simulink model "GOcontroll_Crank_Example"  (R2023b)
settings: Solver=FixedStepDiscrete  StartTime=0.0  StopTime=5  FixedStep=0.01  RelTol=1e-3
PreLoadFcn:
  | librarySetup
PostLoadFcn:
  | core_info = evalc('feature(''numcores'')');
  | core_info_split = split(core_info, " ");
  | num_cores = core_info_split{12};
  | set_param(bdroot, "MakeCommand", ['make_rtw -j' num_cores]);
  | clear num_cores core_info core_info_split
undefined symbols (not defined in the file): DiscIntNeverNeededParam, missing
libraries: GOcontroll_Crank x8, simulink x2
settings Model: Creator=la_obwlf  LastModifiedBy=maud
settings SolverCC: AlgebraicLoopSolver=TrustRegion
settings DataIOCC: LimitDataPoints=on  SaveFormat=Array  ReturnWorkspaceOutputs=off
settings OptimizationCC: BlockReduction=off  DefaultParameterBehavior=Inlined  LifeSpan=1  EfficientTunableParamExpr=on
settings DebuggingCC: SolverPrmCheckMsg=warning  InheritedTsInSrcMsg=none  MultiTaskRateTransMsg=warning  ParameterPrecisionLossMsg=none  UnconnectedInputMsg=warning  UnconnectedOutputMsg=warning  SFUnusedDataAndEventsDiag=none  SFUnexpectedBacktrackingDiag=warning  SFNoUnconditionalDefaultTransitionDiag=warning  SFUndirectedBroadcastEventsDiag=none  SFExecutionAtInitializationDiag=none  RCSCRenamedMsg=none  RCSCObservableMsg=none  ArithmeticOperatorsInVariantConditions=warning
settings HardwareCC: ProdBitPerLong=64  ProdLargestAtomicInteger=Long  ProdLargestAtomicFloat=Double  ProdLongLongMode=on  ProdHWDeviceType=ARM Compatible->ARM 64-bit (LP64)
settings ModelReferenceCC: EnableRefExpFcnMdlSchedulingChecks=on  PropagateSignalLabelsOutOfModel=off
settings SFSimCC: SimUseLocalCustomCode=off  MATLABDynamicMemAlloc=off  CustomCodeUndefinedFunction=UseInterfaceOnly
settings RTWCC: Description=Linux Embedded Coder  SystemTargetFile=ert_linux.tlc  MakeCommand=make_rtw -j24  TemplateMakefile=ert_linux_target_64.tmf  RetainRTWFile=on  RTWUseLocalCustomCode=off
settings CodeAppCC: IgnoreCustomStorageClasses=off  StateflowObjectComments=on
settings STFCustomTargetCC: TargetLangStandard=C89/C90 (ANSI)  CodeReplacementLibrary=GNU C99 extensions  CombineOutputUpdateFcns=on  ERTCustomFileBanners=on  SupportContinuousTime=off  SupportNonInlinedSFcns=off  RemoveResetFunc=on  MATLABClassNameForMDSCustomization=Simulink.SoftwareTarget.ERTCustomization  SystemTargetFile=ert_linux.tlc
settings ERTTargetCC: CodeReplacementLibrary=GNU C99 extensions  MultiwordLength=2048  ParMdlRefBuildCompliant=off  CompOptLevelCompliant=off  ConcurrentExecutionCompliant=off  ModelStepFunctionPrototypeControlCompliant=off  CPPClassGenCompliant=off  UseToolchainInfoCompliant=off  ERTCustomFileTemplate=ert_linux_file_process.tlc  PreserveExpressionOrder=on  SuppressUnreachableDefaultCases=off
settings ConfigComp: CovMetricSettings=dw  CovSaveCumulativeToWorkspaceVar=on  CovSaveSingleToWorkspaceVar=on  CovExternalEMLEnable=off  CovSFcnEnable=off

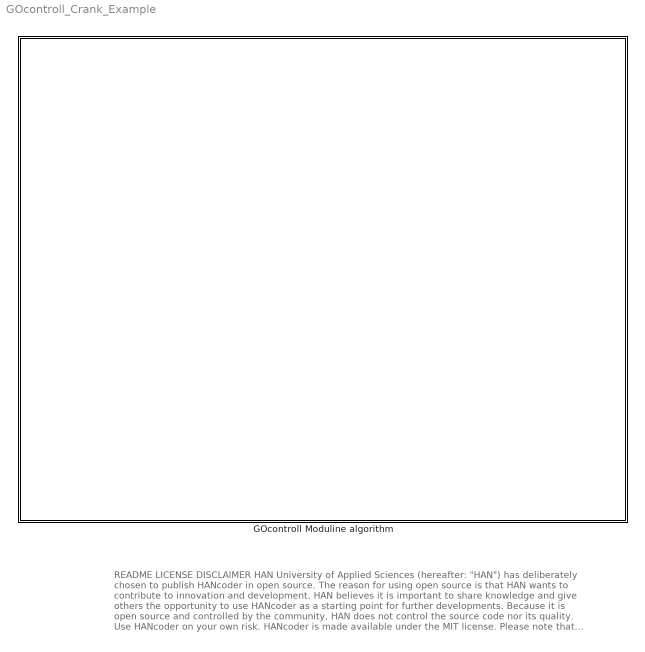
== system GOcontroll_Crank_Example ==
  note: README
      |
      | LICENSE
      |
      | DISCLAIMER
      |
      | HAN University of Applied Sciences (hereafter: "HAN") has deliberately chosen
      | to publish HANcoder in open source. The reason for using open source is that
      | HAN wants to contribute to innovation and development. HAN believes it is
      | important to share knowledge and give others the opportunity to use HANcoder
      | as a starting point for further developments. Because it is open source and
      | controlled by the community, HAN does not control the source code nor its
      | quality. Use HANcoder on your own risk. HANcoder is made available under the
      | MIT license. Please note that this license contains an exclusion of liability.
  GOcontroll Moduline algorithm : Subsystem  mask(TopLevelSubsystem){}
      mask Display: image(imread('GOcontroll.png'))

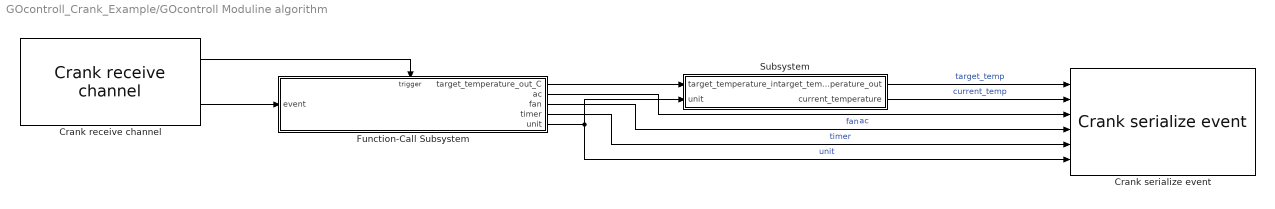
== system GOcontroll_Crank_Example/GOcontroll Moduline algorithm ==
  Crank receive channel : GOcontroll_Crank/Crank receive channel  field_names="[\"num\" \"unit\" string(missing) string(missing) string(missing) string(missing);\"num\" \"unit\" string(missing) string(missing) string(missing) string(missing);\"target_temperature\" \"current_temperature\" \"ac\" \"fan\" \"timer\" \"units\"]"  num_fields=[2 2 6 0 0 0 0]  field_types=[5 5 0 0 0 0;5 5 0 0 0 0;4 4 3 3 3 3]  fmts="[\"2u1 num 2u1 unit\" \"2u1 num 2u1 unit\" \"2s1 target_temperature 2s1 current_temperature 1u1 ac 1u1 fan 1u1 timer 1u1 units\" \"\" \"\" \"\" \"\"]"  tsamp=0.01  nbuff_len=100  channel='thermostat_backend'  header_text=|  events="[\"decrease_temperature\",\"increase_temperature\",\"thermostat_update\",\"toggle_ac\",\"toggle_fan\",\"toggle_timer\",\"toggle_units\"]"  header='ThermostatIO_events.h'  num_events=7
      | #define DECREASE_TEMPERATURE_EVENT "decrease_temperature"
      | #define DECREASE_TEMPERATURE_FMT "2u1 num 2u1 unit"
      | typedef struct {
      | 	uint16_t 		num;
      | 	uint16_t 		unit;
      | } decrease_temperature_event_t;
      | 
      | #define INCREASE_TEMPERATURE_EVENT "increase_temperature"
      | #define INCREASE_TEMPERATURE_FMT "2u1 num 2u1 unit"
      | typedef struct {
      | 	uint16_t 		num;
      | 	uint16_t 		unit;
      | } increase_temperature_event_t;
      | 
      | #define THERMOSTAT_UPDATE_EVENT "thermostat_update"
      | #define THERMOSTAT_UPDATE_FMT "2s1 target_temperature 2s1 current_temperature 1u1 ac 1u1 fan 1u1 timer 1u1 units"
      | typedef struct {
      | 	int16_t 		target_temperature;
      | 	int16_t 		current_temperature;
      | 	uint8_t 		ac;
      | 	uint8_t 		fan;
      | 	uint8_t 		timer;
      | 	uint8_t 		units;
      | } thermostat_update_event_t;
      | 
      | #define TOGGLE_AC_EVENT "toggle_ac"
      | 
      | #define TOGGLE_FAN_EVENT "toggle_fan"
      | 
      | #define TOGGLE_TIMER_EVENT "toggle_timer"
      | 
      | #define TOGGLE_UNITS_EVENT "toggle_units"
      settings: SourceProductName=GOcontroll Crank
  Crank serialize event : GOcontroll_Crank/Crank serialize event  field_types=[5 5 0 0 0 0;5 5 0 0 0 0;4 4 3 3 3 3]  tsamp=0.01  channel='thermostat_frontend'  event_name=thermostat_update  input_names="[\"target_temperature\",\"current_temperature\",\"ac\",\"fan\",\"timer\",\"units\"]"  input_datatypes=[4 4 3 3 3 3]  header='ThermostatIO_events.h'  header_text=|  num_fields=[2 2 6 0 0 0 0]  field_names="[\"num\" \"unit\" string(missing) string(missing) string(missing) string(missing);\"num\" \"unit\" string(missing) string(missing) string(missing) string(missing);\"target_temperature\" \"current_temperature\" \"ac\" \"fan\" \"timer\" \"units\"]"  fmts="[\"2u1 num 2u1 unit\" \"2u1 num 2u1 unit\" \"2s1 target_temperature 2s1 current_temperature 1u1 ac 1u1 fan 1u1 timer 1u1 units\" \"\" \"\" \"\" \"\"]"  events="[\"decrease_temperature\" \"increase_temperature\" \"thermostat_update\" \"toggle_ac\" \"toggle_fan\" \"toggle_timer\" \"toggle_units\"]"
      | #define DECREASE_TEMPERATURE_EVENT "decrease_temperature"
      | #define DECREASE_TEMPERATURE_FMT "2u1 num 2u1 unit"
      | typedef struct {
      | 	uint16_t 		num;
      | 	uint16_t 		unit;
      | } decrease_temperature_event_t;
      | 
      | #define INCREASE_TEMPERATURE_EVENT "increase_temperature"
      | #define INCREASE_TEMPERATURE_FMT "2u1 num 2u1 unit"
      | typedef struct {
      | 	uint16_t 		num;
      | 	uint16_t 		unit;
      | } increase_temperature_event_t;
      | 
      | #define THERMOSTAT_UPDATE_EVENT "thermostat_update"
      | #define THERMOSTAT_UPDATE_FMT "2s1 target_temperature 2s1 current_temperature 1u1 ac 1u1 fan 1u1 timer 1u1 units"
      | typedef struct {
      | 	int16_t 		target_temperature;
      | 	int16_t 		current_temperature;
      | 	uint8_t 		ac;
      | 	uint8_t 		fan;
      | 	uint8_t 		timer;
      | 	uint8_t 		units;
      | } thermostat_update_event_t;
      | 
      | #define TOGGLE_AC_EVENT "toggle_ac"
      | 
      | #define TOGGLE_FAN_EVENT "toggle_fan"
      | 
      | #define TOGGLE_TIMER_EVENT "toggle_timer"
      | 
      | #define TOGGLE_UNITS_EVENT "toggle_units"
      settings: SourceProductName=GOcontroll Crank
  Function-Call Subsystem : Subsystem  TreatAsAtomicUnit=on
  Subsystem : Subsystem
  wires:
  Crank receive channel/1 -> Function-Call Subsystem/Trigger
  Crank receive channel/2 -> Function-Call Subsystem/1(event)
  Function-Call Subsystem/2(ac) -> Crank serialize event/3  "ac"
  Function-Call Subsystem/3(fan) -> Crank serialize event/4  "fan"
  Function-Call Subsystem/4(timer) -> Crank serialize event/5  "timer"
  Function-Call Subsystem/5(unit) -> Subsystem/2(unit), Crank serialize event/6  "unit"
  Subsystem/2(current_temperature) -> Crank serialize event/2  "current_temp"
  Function-Call Subsystem/1(target_temperature_out_C) -> Subsystem/1(target_temperature_in)
  Subsystem/1(target_temperature_out) -> Crank serialize event/1  "target_temp"

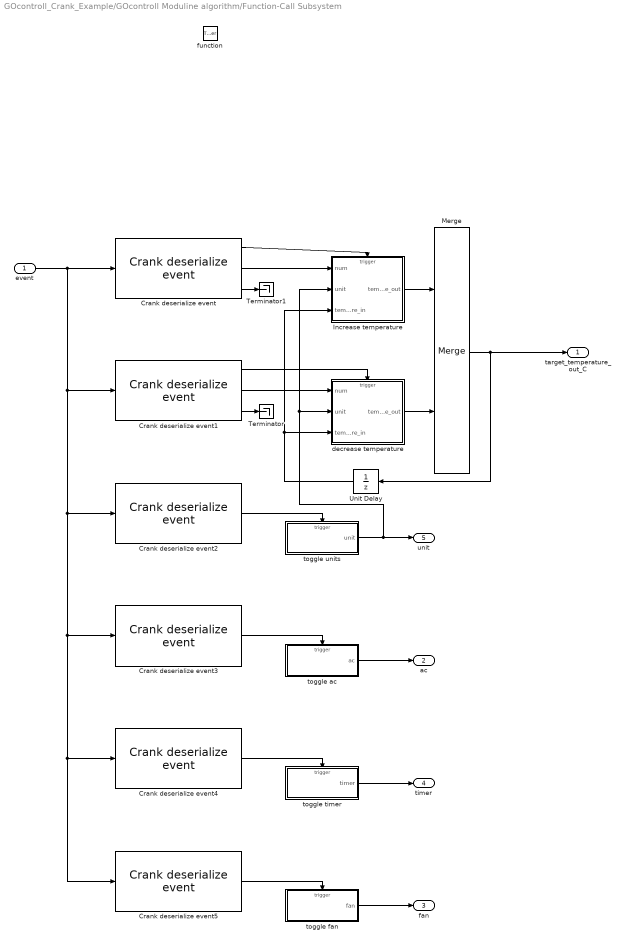
== system GOcontroll_Crank_Example/GOcontroll Moduline algorithm/Function-Call Subsystem ==
  event : Inport
  function : TriggerPort  TriggerType=function-call  VariantControl=(inherit)
  Crank deserialize event : GOcontroll_Crank/Crank deserialize event  channel='thermostat_backend'  event_name=increase_temperature  event_num=1  output_names="[\"num\",\"unit\"]"  output_datatypes=[5 5]
      settings: SourceProductName=GOcontroll Crank
  Crank deserialize event1 : GOcontroll_Crank/Crank deserialize event  channel='thermostat_backend'  event_name=decrease_temperature  event_num=0  output_names="[\"num\",\"unit\"]"  output_datatypes=[5 5]
      settings: SourceProductName=GOcontroll Crank
  Crank deserialize event2 : GOcontroll_Crank/Crank deserialize event  channel='thermostat_backend'  event_name=toggle_units  event_num=6  output_names=[]  output_datatypes=[]
      settings: SourceProductName=GOcontroll Crank
  Crank deserialize event3 : GOcontroll_Crank/Crank deserialize event  channel='thermostat_backend'  event_name=toggle_ac  event_num=3  output_names=[]  output_datatypes=[]
      settings: SourceProductName=GOcontroll Crank
  Crank deserialize event4 : GOcontroll_Crank/Crank deserialize event  channel='thermostat_backend'  event_name=toggle_timer  event_num=5  output_names=[]  output_datatypes=[]
      settings: SourceProductName=GOcontroll Crank
  Crank deserialize event5 : GOcontroll_Crank/Crank deserialize event  channel='thermostat_backend'  event_name=toggle_fan  event_num=4  output_names=[]  output_datatypes=[]
      settings: SourceProductName=GOcontroll Crank
  Increase temperature : Subsystem  TreatAsAtomicUnit=on
  Merge : Merge  InitialOutput=single(16)
  Terminator : Terminator
  Terminator1 : Terminator
  Unit Delay : UnitDelay  InitialCondition=single(16)  SampleTime=-1  HasFrameUpgradeWarning=on
  decrease temperature : Subsystem  TreatAsAtomicUnit=on
  toggle ac : Subsystem  TreatAsAtomicUnit=on
  toggle fan : Subsystem  TreatAsAtomicUnit=on
  toggle timer : Subsystem  TreatAsAtomicUnit=on
  toggle units : Subsystem  TreatAsAtomicUnit=on
  target_temperature_out_C : Outport
  ac : Outport  Port=2
  fan : Outport  Port=3
  timer : Outport  Port=4
  unit : Outport  Port=5
  wires:
  event/1 -> Crank deserialize event5/1, Crank deserialize event4/1, Crank deserialize event3/1, Crank deserialize event2/1, Crank deserialize event1/1, Crank deserialize event/1
  Crank deserialize event/2 -> Increase temperature/1(num)
  Crank deserialize event/1 -> Increase temperature/Trigger
  Crank deserialize event1/1 -> decrease temperature/Trigger
  Crank deserialize event1/2 -> decrease temperature/1(num)
  decrease temperature/1(temperature_out) -> Merge/2
  Increase temperature/1(temperature_out) -> Merge/1
  Crank deserialize event2/1 -> toggle units/Trigger
  toggle units/1(unit) -> Increase temperature/2(unit), decrease temperature/2(unit), unit/1
  Crank deserialize event3/1 -> toggle ac/Trigger
  toggle ac/1(ac) -> ac/1
  toggle timer/1(timer) -> timer/1
  Crank deserialize event4/1 -> toggle timer/Trigger
  Crank deserialize event5/1 -> toggle fan/Trigger
  toggle fan/1(fan) -> fan/1
  Unit Delay/1 -> Increase temperature/3(temperature_in), decrease temperature/3(temperature_in)
  Merge/1 -> Unit Delay/1, target_temperature_out_C/1
  Crank deserialize event1/3 -> Terminator/1
  Crank deserialize event/3 -> Terminator1/1

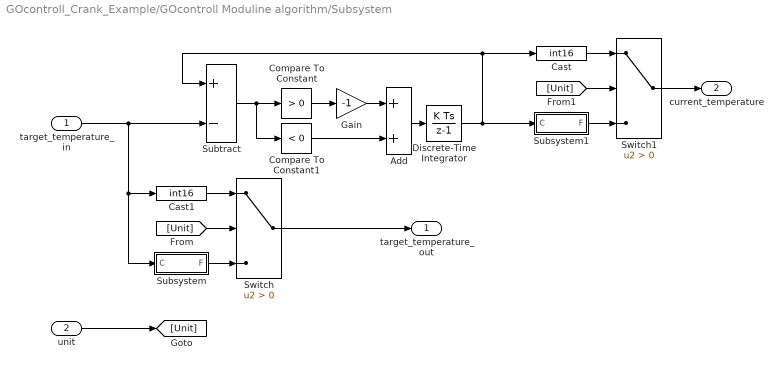
== system GOcontroll_Crank_Example/GOcontroll Moduline algorithm/Subsystem ==
  target_temperature_in : Inport
  unit : Inport  Port=2
  Add : Sum  OutDataTypeStr=int16  AccumDataTypeStr=int16
  Cast : DataTypeConversion  OutDataTypeStr=int16  SaturateOnIntegerOverflow=off  RndMeth=Floor
  Cast1 : DataTypeConversion  OutDataTypeStr=int16  SaturateOnIntegerOverflow=off  RndMeth=Floor
  Compare To Constant : simulink/Logic and Bit Operations/Compare To Constant  relop=>  const=0  OutDataTypeStr=uint8
  Compare To Constant1 : simulink/Logic and Bit Operations/Compare To Constant  relop=<  const=0  OutDataTypeStr=uint8
  Discrete-Time Integrator : DiscreteIntegrator  gainval=0.5  InitialCondition=16  SampleTime=2  OutDataTypeStr=single  ICPrevOutput=DiscIntNeverNeededParam  ICPrevScaledInput=DiscIntNeverNeededParam
  Gain : Gain  Gain=-1  ParamDataTypeStr=int16  OutDataTypeStr=single
  Subsystem : Subsystem
  Subsystem1 : Subsystem
  Subtract : Sum  Inputs=+-
  Switch : Switch  Criteria=u2 > Threshold  SaturateOnIntegerOverflow=off  InputSameDT=off
  Switch1 : Switch  Criteria=u2 > Threshold  SaturateOnIntegerOverflow=off  InputSameDT=off
  target_temperature_out : Outport
  current_temperature : Outport  Port=2
  wires:
  Subtract/1 -> Compare To Constant1/1, Compare To Constant/1
  Compare To Constant/1 -> Gain/1
  Gain/1 -> Add/1
  Compare To Constant1/1 -> Add/2
  Add/1 -> Discrete-Time Integrator/1
  Switch/1 -> target_temperature_out/1
  Subsystem/1(F) -> Switch/3
  target_temperature_in/1 -> Subsystem/1(C), Cast1/1, Subtract/2
  [Unit] -> Switch/2
  unit/1 -> [Unit]
  [Unit] -> Switch1/2
  Discrete-Time Integrator/1 -> Subsystem1/1(C), Cast/1, Subtract/1
  Subsystem1/1(F) -> Switch1/3
  Switch1/1 -> current_temperature/1
  Cast/1 -> Switch1/1
  Cast1/1 -> Switch/1

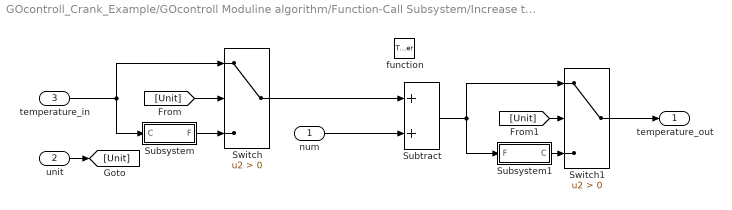
== system GOcontroll_Crank_Example/GOcontroll Moduline algorithm/Function-Call Subsystem/Increase temperature ==
  num : Inport
  unit : Inport  Port=2
  temperature_in : Inport  Port=3  Unit=degC
  function : TriggerPort  TriggerType=function-call  VariantControl=(inherit)
  Subsystem : Subsystem
  Subsystem1 : Subsystem
  Subtract : Sum  OutDataTypeStr=single  AccumDataTypeStr=single
  Switch : Switch  Criteria=u2 > Threshold  SaturateOnIntegerOverflow=off  InputSameDT=off
  Switch1 : Switch  Criteria=u2 > Threshold  SaturateOnIntegerOverflow=off  InputSameDT=off
  temperature_out : Outport  InitialOutput=single(16)
  wires:
  Switch/1 -> Subtract/1
  num/1 -> Subtract/2
  [Unit] -> Switch/2
  unit/1 -> [Unit]
  [Unit] -> Switch1/2
  Subtract/1 -> Subsystem1/1(F), Switch1/1
  Switch1/1 -> temperature_out/1
  Subsystem/1(F) -> Switch/3
  temperature_in/1 -> Subsystem/1(C), Switch/1
  Subsystem1/1(C) -> Switch1/3

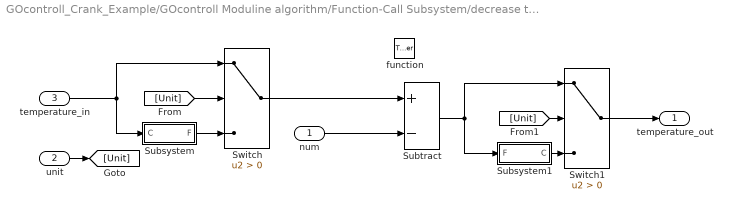
== system GOcontroll_Crank_Example/GOcontroll Moduline algorithm/Function-Call Subsystem/decrease temperature ==
  num : Inport
  unit : Inport  Port=2
  temperature_in : Inport  Port=3  Unit=degC
  function : TriggerPort  TriggerType=function-call  VariantControl=(inherit)
  Subsystem : Subsystem
  Subsystem1 : Subsystem
  Subtract : Sum  Inputs=+-  OutDataTypeStr=single  AccumDataTypeStr=single
  Switch : Switch  Criteria=u2 > Threshold  SaturateOnIntegerOverflow=off  InputSameDT=off
  Switch1 : Switch  Criteria=u2 > Threshold  SaturateOnIntegerOverflow=off  InputSameDT=off
  temperature_out : Outport  InitialOutput=int16(16)
  wires:
  num/1 -> Subtract/2
  temperature_in/1 -> Subsystem/1(C), Switch/1
  Subtract/1 -> Subsystem1/1(F), Switch1/1
  unit/1 -> [Unit]
  [Unit] -> Switch/2
  Switch/1 -> Subtract/1
  [Unit] -> Switch1/2
  Switch1/1 -> temperature_out/1
  Subsystem/1(F) -> Switch/3
  Subsystem1/1(C) -> Switch1/3

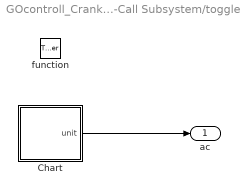
== system GOcontroll_Crank_Example/GOcontroll Moduline algorithm/Function-Call Subsystem/toggle ac ==
  function : TriggerPort  TriggerType=function-call  VariantControl=(inherit)
  Chart : Stateflow chart  TreatAsAtomicUnit=on
  ac : Outport
  wires:
  Chart/1(unit) -> ac/1

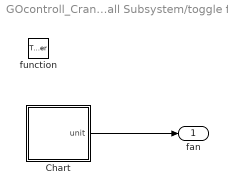
== system GOcontroll_Crank_Example/GOcontroll Moduline algorithm/Function-Call Subsystem/toggle fan ==
  function : TriggerPort  TriggerType=function-call  VariantControl=(inherit)
  Chart : Stateflow chart  TreatAsAtomicUnit=on
  fan : Outport
  wires:
  Chart/1(unit) -> fan/1

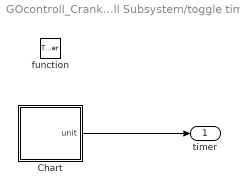
== system GOcontroll_Crank_Example/GOcontroll Moduline algorithm/Function-Call Subsystem/toggle timer ==
  function : TriggerPort  TriggerType=function-call  VariantControl=(inherit)
  Chart : Stateflow chart  TreatAsAtomicUnit=on
  timer : Outport
  wires:
  Chart/1(unit) -> timer/1

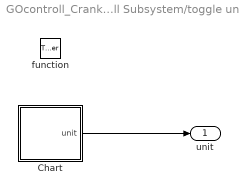
== system GOcontroll_Crank_Example/GOcontroll Moduline algorithm/Function-Call Subsystem/toggle units ==
  function : TriggerPort  TriggerType=function-call  VariantControl=(inherit)
  Chart : Stateflow chart  TreatAsAtomicUnit=on
  unit : Outport
  wires:
  Chart/1(unit) -> unit/1

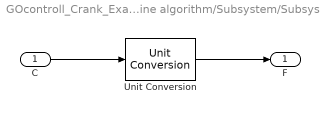
== system GOcontroll_Crank_Example/GOcontroll Moduline algorithm/Subsystem/Subsystem ==
  C : Inport  Unit=degC
  Unit Conversion : UnitConversion  OutputType=Inherit: Inherit via back propagation
  F : Outport  OutDataTypeStr=int16  Unit=degF
  wires:
  C/1 -> Unit Conversion/1
  Unit Conversion/1 -> F/1

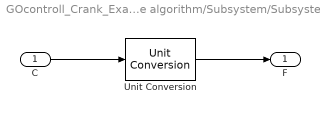
== system GOcontroll_Crank_Example/GOcontroll Moduline algorithm/Subsystem/Subsystem1 ==
  C : Inport  Unit=degC
  Unit Conversion : UnitConversion  OutputType=Inherit: Inherit via back propagation
  F : Outport  OutDataTypeStr=int16  Unit=degF
  wires:
  Unit Conversion/1 -> F/1
  C/1 -> Unit Conversion/1

== system GOcontroll_Crank_Example/GOcontroll Moduline algorithm/Function-Call Subsystem/Increase temperature/Subsystem ==
  C : Inport  Unit=degC
  Unit Conversion : UnitConversion  OutputType=Inherit: Inherit via back propagation
  F : Outport  OutDataTypeStr=single  Unit=degF
  wires:
  C/1 -> Unit Conversion/1
  Unit Conversion/1 -> F/1

== system GOcontroll_Crank_Example/GOcontroll Moduline algorithm/Function-Call Subsystem/Increase temperature/Subsystem1 ==
  F : Inport  Unit=degF
  Unit Conversion : UnitConversion  OutputType=Inherit: Inherit via back propagation
  C : Outport  OutDataTypeStr=single  Unit=degC
  wires:
  Unit Conversion/1 -> C/1
  F/1 -> Unit Conversion/1

== system GOcontroll_Crank_Example/GOcontroll Moduline algorithm/Function-Call Subsystem/decrease temperature/Subsystem ==
  C : Inport  Unit=degC
  Unit Conversion : UnitConversion  OutputType=Inherit: Inherit via back propagation
  F : Outport  OutDataTypeStr=single  Unit=degF
  wires:
  C/1 -> Unit Conversion/1
  Unit Conversion/1 -> F/1

== system GOcontroll_Crank_Example/GOcontroll Moduline algorithm/Function-Call Subsystem/decrease temperature/Subsystem1 ==
  F : Inport  Unit=degF
  Unit Conversion : UnitConversion  OutputType=Inherit: Inherit via back propagation
  C : Outport  OutDataTypeStr=single  Unit=degC
  wires:
  Unit Conversion/1 -> C/1
  F/1 -> Unit Conversion/1

== stateflow chart GOcontroll_Crank_Example/GOcontroll Moduline algorithm/Function-Call Subsystem/toggle ac/Chart ==
  state celsius
    en: unit = 1;
  state fahrenheit
    en: unit = 0;
  (default) -> celsius
  celsius -> fahrenheit
  fahrenheit -> celsius
  data: unit output uint8 =uint8(0)

== stateflow chart GOcontroll_Crank_Example/GOcontroll Moduline algorithm/Function-Call Subsystem/toggle units/Chart ==
  state fahrenheit1
    en: unit = 0;
  state celsius
    en: unit = 1;
  (default) -> fahrenheit1
  fahrenheit1 -> celsius
  celsius -> fahrenheit1
  data: unit output uint8 =uint8(1)

== stateflow chart GOcontroll_Crank_Example/GOcontroll Moduline algorithm/Function-Call Subsystem/toggle fan/Chart ==
  state celsius
    en: unit = 1;
  state fahrenheit
    en: unit = 0;
  (default) -> celsius
  celsius -> fahrenheit
  fahrenheit -> celsius
  data: unit output uint8 =uint8(0)

== stateflow chart GOcontroll_Crank_Example/GOcontroll Moduline algorithm/Function-Call Subsystem/toggle timer/Chart ==
  state celsius
    en: unit = 1;
  state fahrenheit
    en: unit = 0;
  (default) -> celsius
  celsius -> fahrenheit
  fahrenheit -> celsius
  data: unit output uint8 =uint8(0)
